simulink model "asbCubeSat.backup_210716a"  (R2020b)
settings: Solver=ode3  StartTime=0.0  StopTime=stopTime  FixedStep=CubeSatTimeStep  RelTol=1e-3  EnableMultiTasking=on
PreLoadFcn:
  | if ~builtin('license','test','Virtual_Reality_Toolbox')
  |     assignin('base','variantVisualization',0)
  | end
InitFcn:
  | if evalin('base', 'exist(''variantVisualization'',''var'')') && ...
  |         evalin('base', 'variantVisualization == 1')
  |     if ~builtin('license','checkout','Virtual_Reality_Toolbox')
  |         error(message('aeroblks_cubesat:cubesat:licenseFailAnim'));
  |     end
  | end
  | 
  | if ~evalin('base','exist(''CubeSatTimeStep'')')
  |     assignin('base','CubeSatTimeStep',1);
  | end
libraries: aerolibutil x20, aerolibconvert2 x7, simulink x3, vrlib x2, asbCubeSatEnvironmentLib x1, SignalEditorBlockLib x1, sharedutil x1, asbCubeSatActuatorsLib x1, asbCubeSatSensorsLib x1, asbCubeSatDynamicsLib x1, asbCubeSatFSWLib x1, aerolibobsolete x1
settings Model: RequirementInfo={} %GIDa_aedc6be2_fb6a_446c_8c25_10b8bc9db182  SnapshotInterval=1  EnablePacing=on  PacingRate=333  ExtModeAutoUpdateStatusClock=off  OrderedModelArguments=off  Creator=The MathWorks, Inc.  LastModifiedBy=Rodrigo.weber
settings DataIOCC: LimitDataPoints=on  SaveFormat=Array  SaveOutput=off  DSMLogging=off  SaveTime=off  ReturnWorkspaceOutputs=off
settings OptimizationCC: DefaultParameterBehavior=Inlined  OptimizeBlockIOStorage=off  BufferReuse=off  GlobalBufferReuse=off  ExpressionFolding=off  ExpressionDepthLimit=2147483647  LocalBlockOutputs=off  InitFltsAndDblsToZero=on  LifeSpan=inf  OptimizeDataStoreBuffers=off  BusAssignmentInplaceUpdate=off
settings DebuggingCC: SignalResolutionControl=TryResolveAllWithWarning  MultiTaskDSMMsg=warning  MultiTaskCondExecSysMsg=none  AssertControl=DisableAll  StateNameClashWarn=warning  PregeneratedLibrarySubsystemCodeDiagnostic=none  SFUnexpectedBacktrackingDiag=warning  SFNoUnconditionalDefaultTransitionDiag=warning  SFExecutionAtInitializationDiag=none  ArithmeticOperatorsInVariantConditions=warning
settings HardwareCC: ProdBitPerPointer=32  ProdBitPerSizeT=32  ProdBitPerPtrDiffT=32  ProdLargestAtomicFloat=None  ProdIntDivRoundTo=Undefined  ProdEndianess=Unspecified  ProdWordSize=32  ProdHWDeviceType=32-bit Generic
settings ModelReferenceCC: UpdateModelReferenceTargets=IfOutOfDate  ModelReferenceMinAlgLoopOccurrences=on  PropagateSignalLabelsOutOfModel=off
settings SFSimCC: SimUseLocalCustomCode=off
settings RTWCC: RTWUseLocalCustomCode=off
settings CodeAppCC: StateflowObjectComments=on
settings GRTTargetCC: TargetFcnLib=ansi_tfl_tmw.mat  TargetLangStandard=C89/C90 (ANSI)  CombineOutputUpdateFcns=off  GRTInterface=on
settings ConfigComp: CovMetricSettings=dw  CovSaveCumulativeToWorkspaceVar=on  CovSaveSingleToWorkspaceVar=on  CovExternalEMLEnable=off

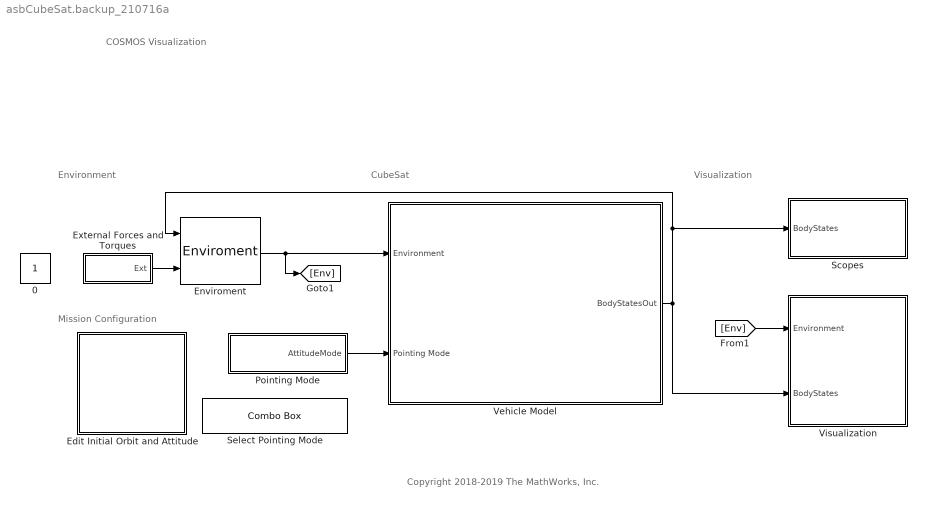
== system asbCubeSat.backup_210716a ==
  note: Visualization
  note: CubeSat
  note: Environment
  note: Copyright 2018-2019 The MathWorks, Inc.
  note: COSMOS
      | Visualization
  note: Mission Configuration
  Edit Initial Orbit and Attitude : Subsystem  mask(CubeSat Initial Conditions){sim_t0=2458488, epoch=2451545, method=Keplerian Orbital Elements, a=7086233.13, ecc=0, incl=51.7519, omega=95.2562, argp=93.4872, nu=302.9234, truelon=0, arglat=0, lonper=0, r_eci=[-649165.38524 7056435.6637 0], v_eci=[-4623.4845 -425.34309 5890.0297], r_ecef=[-7011830.8459 1024171.027 -1366.7752123], v_ecef=[-599.03035 -4093.3209 5881.6205], lla=[-0.01111806026 171.6899547 708096.1308], v_ned=[5881.6206 4136.9206 0.0068768912], euler=[0 0 0], pqr=[0 0 -0.05168], dAT=37, dUT1=-0.1193, pm=[2.141e-05 6.93e-05], dCIP=[1.014e-07 -6.81e-08], lod=0}
      mask prompts: sim_t0 "aeroblks_cubesat:cubesat:StartDate"; epoch "aeroblks_cubesat:cubesat:ECIEpoch"; method "aeroblks_cubesat:cubesat:InputMethod"; a "aeroblks_cubesat:cubesat:SemiMajorAxis"; ecc "aeroblks_cubesat:cubesat:Eccentricity"; incl "aeroblks_cubesat:cubesat:Inclination"; omega "aeroblks_cubesat:cubesat:RAAN"; argp "aeroblks_cubesat:cubesat:ArgP"; nu "aeroblks_cubesat:cubesat:TrueAnomaly"; truelon "aeroblks_cubesat:cubesat:TrueLon"; arglat "aeroblks_cubesat:cubesat:ArgLat"; lonper "aeroblks_cubesat:cubesat:LonPer"; r_eci "aeroblks_cubesat:cubesat:ECIPos"; v_eci "aeroblks_cubesat:cubesat:ECIVel"; r_ecef "aeroblks_cubesat:cubesat:ECEFPos"; v_ecef "aeroblks_cubesat:cubesat:ECEFVel"; lla "aeroblks_cubesat:cubesat:LLA"; v_ned "aeroblks_cubesat:cubesat:NEDVel"; euler "aeroblks_cubesat:cubesat:Euler"; pqr "aeroblks_cubesat:cubesat:BodyAngRates"; dAT "aeroblks_cubesat:cubesat:dTAI"; dUT1 "aeroblks_cubesat:cubesat:DUT1"; pm "aeroblks_cubesat:cubesat:DPolar"; dCIP "aeroblks_cubesat:cubesat:DCIP"; lod "aeroblks_cubesat:cubesat:DLOD"
      mask help: aeroblks_cubesat:cubesat:InitCondBlockDesc
      mask init:
      | initCond = cubeSatCallback(gcb, 'computeIC', method, sim_t0, epoch, a, ecc, incl,...
      |     omega, argp, nu, truelon, arglat, lonper, r_eci, v_eci, r_ecef, v_ecef, lla,...
      |     v_ned, euler, pqr, dAT, dUT1, pm, dCIP, lod);
      mask TypeOptions method: aeroblks_cubesat:cubesat:InputKeplerian | aeroblks_cubesat:cubesat:InputECI | aeroblks_cubesat:cubesat:InputECEF | aeroblks_cubesat:cubesat:InputLLANED
      mask Callback method: cubeSatCallback(gcb, 'handleMethod');
      mask Callback ecc: cubeSatCallback(gcb, 'handleCircularOrbit');
      mask Callback incl: cubeSatCallback(gcb, 'handleCircularOrbit');
      mask DialogControl sim_t0 Prompt: Start date [Julian date]:
      mask DialogControl sim_t0 Tooltip: aeroblks_cubesat:cubesat:StartDateTT
      mask DialogControl icTab Prompt: aeroblks_cubesat:cubesat:InitCond
      mask DialogControl epoch Prompt: Epoch of ECI frame [Julian date]:
      mask DialogControl epoch Tooltip: aeroblks_cubesat:cubesat:ECIEpochTT
      mask DialogControl Container9 Prompt: aeroblks_cubesat:cubesat:InitCondOrbit
      mask DialogControl method Prompt: Input method:
      mask DialogControl method Tooltip: aeroblks_cubesat:cubesat:InputMethodTT
      mask DialogControl a Prompt: Semi-major axis [m]:
      mask DialogControl a Tooltip: aeroblks_cubesat:cubesat:SemiMajorAxisTT
      mask DialogControl ecc Prompt: Eccentricity:
      mask DialogControl ecc Tooltip: aeroblks_cubesat:cubesat:EccentricityTT
      mask DialogControl incl Prompt: Inclination [deg]:
      mask DialogControl incl Tooltip: aeroblks_cubesat:cubesat:InclinationTT
      mask DialogControl omega Prompt: Right ascension of the ascending node [deg]:
      mask DialogControl omega Tooltip: aeroblks_cubesat:cubesat:RAANTT
      mask DialogControl argp Prompt: Argument of periapsis [deg]:
      mask DialogControl argp Tooltip: aeroblks_cubesat:cubesat:ArgPTT
      mask DialogControl nu Prompt: True anomaly [deg]:
      mask DialogControl nu Tooltip: aeroblks_cubesat:cubesat:TrueAnomalyTT
      mask DialogControl truelon Prompt: True longitude [deg] (circular equatorial):
      mask DialogControl truelon Tooltip: aeroblks_cubesat:cubesat:TrueLonTT
      mask DialogControl arglat Prompt: Argument of latitude [deg] (circular inclined):
      mask DialogControl arglat Tooltip: aeroblks_cubesat:cubesat:ArgLatTT
      mask DialogControl lonper Prompt: Longitude of periapsis [deg] (elliptical equatorial):
      mask DialogControl lonper Tooltip: aeroblks_cubesat:cubesat:LonPerTT
      mask DialogControl r_eci Prompt: ECI position vector [m]:
      mask DialogControl r_eci Tooltip: aeroblks_cubesat:cubesat:ECIPosTT
      mask DialogControl v_eci Prompt: ECI velocity vector [m/s]:
      mask DialogControl v_eci Tooltip: aeroblks_cubesat:cubesat:ECIVelTT
      mask DialogControl r_ecef Prompt: ECEF position vector [m]:
      mask DialogControl r_ecef Tooltip: aeroblks_cubesat:cubesat:ECEFPosTT
      mask DialogControl v_ecef Prompt: ECEF velocity vector [m/s]:
      mask DialogControl v_ecef Tooltip: aeroblks_cubesat:cubesat:ECEFVelTT
      mask DialogControl lla Prompt: Geodetic latitude, longitude, altitude [deg, deg, m]:
      mask DialogControl lla Tooltip: aeroblks_cubesat:cubesat:LLATT
      mask DialogControl v_ned Prompt: NED velocity vector [m/s]:
      mask DialogControl v_ned Tooltip: aeroblks_cubesat:cubesat:NEDVelTT
      mask DialogControl Container11 Prompt: aeroblks_cubesat:cubesat:InitCondAttitude
      mask DialogControl euler Prompt: <html>Initial Euler angles (roll, pitch, yaw) [deg]:</html>
      mask DialogControl euler Tooltip: aeroblks_cubesat:cubesat:EulerTT
      mask DialogControl pqr Prompt: Initial body angular rates [deg/s]:
      mask DialogControl pqr Tooltip: aeroblks_cubesat:cubesat:BodyAngRatesTT
      mask DialogControl epTab Prompt: aeroblks_cubesat:cubesat:EOPTab
      mask DialogControl dAT Prompt: Difference between TAI and UTC [sec]:
      mask DialogControl dAT Tooltip: aeroblks_cubesat:cubesat:dTAITT
      mask DialogControl dUT1 Prompt: Difference between UTC and UT1 [sec]:
      mask DialogControl dUT1 Tooltip: aeroblks_cubesat:cubesat:DUT1TT
      mask DialogControl pm Prompt: Polar displacement [deg deg]:
      mask DialogControl pm Tooltip: aeroblks_cubesat:cubesat:DPolarTT
      mask DialogControl dCIP Prompt: CIP adjustment [deg deg]:
      mask DialogControl dCIP Tooltip: aeroblks_cubesat:cubesat:DCIPTT
      mask DialogControl lod Prompt: Excess length of day [sec]:
      mask DialogControl lod Tooltip: aeroblks_cubesat:cubesat:DLODTT
      mask Display:
      | text(.1, .9, [' a = ' sprintf('%.1f', str2double(get_param(gcb, 'a'))) ' m'],'horizontalAlignment','left','texmode','on');
      | text(.1, .75, [' e = ' get_param(gcb, 'ecc')],'horizontalAlignment','left','texmode', 'on')
      | text(.1, .6, ['  i = ' get_param(gcb, 'incl') '\circ'],'horizontalAlignment','left','texmode', 'on')
      | text(.1, .45, ['\Omega = ' get_param(gcb, 'omega') '\circ'],'horizontalAlignment','left','texmode', 'on')
      | text(.1, .3, ['\omega = ' get_param(gcb, 'argp') '\circ'],'horizontalAlignment','left','texmode', 'on')
      | text(.1, .15, [' \nu = ' get_param(gcb, 'nu') '\circ'],'horizontalAlignment','left','texmode', 'on')
  Enviroment : asbCubeSatEnvironmentLib/Enviroment  SystemSampleTime=-1  VariantActivationTime=update diagram  Latency=0  AutoFrameSizeCalculation=off
  "External Forces and Torques " : Subsystem
  Pointing Mode : Subsystem
  Scopes : Subsystem  VariantControl=visOff
  Select Pointing Mode : ComboBox  LabelPosition=Hide  SelectedLabel=Nadir Pointing (Earth)
      settings: Values={{'Standby', 'Nadir Pointing (Earth)', 'Sun Tracking', 'Custom Schedule'}, [0 1 2 3]}
  Vehicle Model : Subsystem
      mask Display: image('CubeSatVehicle.PNG');
  Visualization : Subsystem  Variant=on  mask(Set Animation Properties){visSampleTime=5, cubesatSize=2e5, showAntenna=on, antennaHeight=1e6, antennaHalfAngle=25}
      mask prompts: visSampleTime "aeroblks_cubesat:cubesat:AnimSampleTime"; cubesatSize "aeroblks_cubesat:cubesat:MdlSize"; showAntenna "aeroblks_cubesat:cubesat:ShowCone"; antennaHeight "aeroblks_cubesat:cubesat:ConeHeight"; antennaHalfAngle "aeroblks_cubesat:cubesat:ConeAngle"
      mask help: aeroblks_cubesat:cubesat:VisBlockDesc
      mask Callback showAntenna:
      | if evalin('base', 'exist(''variantVisualization'',''var'')') ...
      |     && evalin('base', 'variantVisualization == 1') ...
      |     && builtin('license','test','Virtual_Reality_Toolbox')
      | 
      |     enable = get_param(gcb,'MaskEnables');
      |     if strcmp(get_param(gcb, 'showAntenna'), 'off')
      |         enable(4:5) = {'off'};
      |     else
      |         enable(4:5) = {'on'};
      |     end
      |     set_param(gcb,'MaskEnables', enable);
      |     clear enable
      | end
      mask DialogControl vrOpenBtn Prompt: aeroblks_cubesat:cubesat:AnimOpenBtn
      mask DialogControl vrOpenBtn Callback:
      | if builtin('license','checkout','Virtual_Reality_Toolbox')
      |     vrmfunc('FnOpen',getSimulinkBlockHandle([gcb '/Virtual Reality World/VR Sink']));
      | end
      mask DialogControl visSampleTime Prompt: Animation refresh rate:
      mask DialogControl visSampleTime Tooltip: aeroblks_cubesat:cubesat:AnimSampleTimeTT
      mask DialogControl cubesatSize Prompt: CubeSat display size [m]:
      mask DialogControl cubesatSize Tooltip: aeroblks_cubesat:cubesat:MdlSizeTT
      mask DialogControl Container3 Prompt: aeroblks_cubesat:cubesat:AntennaPropArea
      mask DialogControl showAntenna Prompt: Show antenna cone in animation
      mask DialogControl showAntenna Tooltip: aeroblks_cubesat:cubesat:ShowConeTT
      mask DialogControl antennaHeight Prompt: Antenna cone height [m]:
      mask DialogControl antennaHeight Tooltip: aeroblks_cubesat:cubesat:ConeHeightTT
      mask DialogControl antennaHalfAngle Prompt: Antenna cone half angle [deg]:
      mask DialogControl antennaHalfAngle Tooltip: aeroblks_cubesat:cubesat:ConeAngleTT
  0 : Constant  IOType=siggen
  wires:
  Enviroment/1 -> [Env], Vehicle Model/1(Environment)
  "External Forces and Torques "/1(Ext) -> Enviroment/2
  Vehicle Model/1(BodyStatesOut) -> Visualization/2(BodyStates), Scopes/1(BodyStates), Enviroment/1
  Pointing Mode/1(AttitudeMode) -> Vehicle Model/2(Pointing Mode)
  [Env] -> Visualization/1(Environment)

== system asbCubeSat.backup_210716a/Edit Initial Orbit and Attitude ==

== system asbCubeSat.backup_210716a/External Forces and Torques  ==
  Forces_Body : Constant  Value=[0 0 0]
  Mux : Mux  RequirementInfo={} %GIDa_ef4ca723_4eef_40f8_bb1e_99de60d2b248  Inputs=2
  Torques_Body : Constant  Value=[0 0 0]
  Ext : Outport  RequirementInfo={} %GIDa_0f078eca_6127_499d_b81c_658503a40261  VectorParamsAs1DForOutWhenUnconnected=off
  wires:
  Forces_Body/1 -> Mux/1
  Torques_Body/1 -> Mux/2
  Mux/1 -> Ext/1

== system asbCubeSat.backup_210716a/Pointing Mode ==
  note: Modes:
      | 0 = Off
      | 1 = Earth (Nadir)
      | 2 = Sun
  Mode : Constant  SampleTime=-1
  Multiport Switch : MultiPortSwitch  DataPortOrder=Specify indices  DataPortIndices={3, [0,1,2]}  DiagnosticForDefault=None
  Signal Editor : SignalEditorBlockLib/Signal Editor  FileName=SignalEditorPointing.mat  ActiveScenario=PointingScenario  ActiveSignal=PointingMode  IsBus=off  OutputBusObjectStr=Bus: BusObject  SampleTime=0  Interpolate=off  ZeroCross=off  OutputAfterFinalValue=Setting to zero  Unit=inherit  PreserveSignalName=on
  AttitudeMode : Outport  VectorParamsAs1DForOutWhenUnconnected=off
  wires:
  Signal Editor/1 -> Multiport Switch/2
  Mode/1 -> Multiport Switch/1, Multiport Switch/3
  Multiport Switch/1 -> AttitudeMode/1

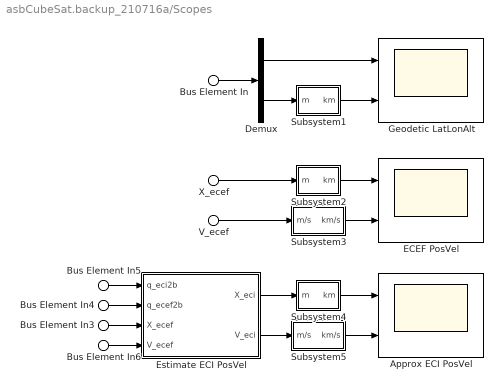
== system asbCubeSat.backup_210716a/Scopes ==
  Bus Element In : Inport  PortName=BodyStates  Element=LatLonAlt
  X_ecef : Inport  PortName=BodyStates  Element=X_ecef
  Bus Element In3 : Inport  PortName=BodyStates  Element=X_ecef
  V_ecef : Inport  PortName=BodyStates  Element=V_ecef
  Bus Element In6 : Inport  PortName=BodyStates  Element=V_ecef
  Bus Element In4 : Inport  PortName=BodyStates  Element=q_ecef2b
  Bus Element In5 : Inport  PortName=BodyStates  Element=q_eci2b
  Approx ECI PosVel : Scope  NumInputPorts=2
  Demux : Demux  Outputs=[2 1]
  ECEF PosVel : Scope  NumInputPorts=2
  Estimate ECI PosVel : Subsystem
  Geodetic LatLonAlt : Scope  NumInputPorts=2
  Subsystem1 : Subsystem
  Subsystem2 : Subsystem
  Subsystem3 : Subsystem
  Subsystem4 : Subsystem
  Subsystem5 : Subsystem
  wires:
  Bus Element In/1 -> Demux/1
  Demux/1 -> Geodetic LatLonAlt/1
  Demux/2 -> Subsystem1/1(m)
  X_ecef/1 -> Subsystem2/1(m)
  V_ecef/1 -> Subsystem3/1(m/s)
  Estimate ECI PosVel/1(X_eci) -> Subsystem4/1(m)
  Estimate ECI PosVel/2(V_eci) -> Subsystem5/1(m/s)
  Bus Element In5/1 -> Estimate ECI PosVel/1(q_eci2b)
  Bus Element In4/1 -> Estimate ECI PosVel/2(q_ecef2b)
  Bus Element In3/1 -> Estimate ECI PosVel/3(X_ecef)
  Bus Element In6/1 -> Estimate ECI PosVel/4(V_ecef)
  Subsystem1/1(km) -> Geodetic LatLonAlt/2
  Subsystem2/1(km) -> ECEF PosVel/1
  Subsystem3/1(km/s) -> ECEF PosVel/2
  Subsystem4/1(km) -> Approx ECI PosVel/1
  Subsystem5/1(km/s) -> Approx ECI PosVel/2

== system asbCubeSat.backup_210716a/Vehicle Model ==
  note: Flight Software
  note: Plant Model
  Environment : Inport
  Pointing Mode : Inport  Port=2
  Vehicle Control Actuators : asbCubeSatActuatorsLib/Vehicle Control Actuators  SystemSampleTime=-1  VariantActivationTime=update diagram  Latency=0  AutoFrameSizeCalculation=off
  Vehicle Control Sensors : asbCubeSatSensorsLib/Vehicle Control Sensors  SystemSampleTime=-1  VariantActivationTime=update diagram  Latency=0  AutoFrameSizeCalculation=off
  Vehicle Dynamics : asbCubeSatDynamicsLib/Vehicle Dynamics  SystemSampleTime=-1  VariantActivationTime=update diagram  Latency=0  AutoFrameSizeCalculation=off
  Vehicle Flight Software : asbCubeSatFSWLib/Vehicle Flight Software  SystemSampleTime=-1  VariantActivationTime=update diagram  Latency=0  AutoFrameSizeCalculation=off
  BodyStatesOut : Outport  OutDataTypeStr=Bus: StatesOutBus  VectorParamsAs1DForOutWhenUnconnected=off
  wires:
  Vehicle Dynamics/1 -> Vehicle Control Sensors/1, BodyStatesOut/1
  Pointing Mode/1 -> Vehicle Flight Software/1
  Vehicle Control Sensors/1 -> Vehicle Flight Software/3
  Vehicle Control Actuators/1 -> Vehicle Dynamics/1
  Vehicle Control Actuators/2 -> Vehicle Dynamics/2
  Vehicle Flight Software/1 -> Vehicle Control Actuators/1
  Environment/1 -> Vehicle Dynamics/3, Vehicle Flight Software/2

== system asbCubeSat.backup_210716a/Visualization ==
  Environment : Inport
  BodyStates : Inport  RequirementInfo={} %GIDa_d1e0371a_f352_4707_a071_6ff04189e700  Port=2
  No Visualization : Subsystem  VariantControl=visOff
  Virtual Reality World : Subsystem  VariantControl=visSL3D

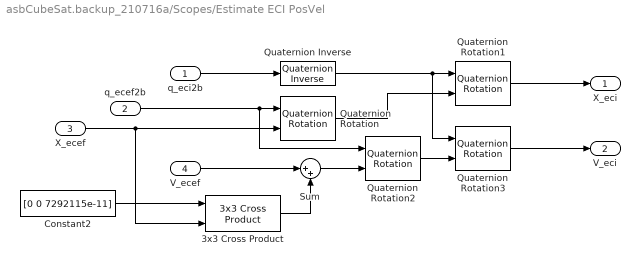
== system asbCubeSat.backup_210716a/Scopes/Estimate ECI PosVel ==
  q_eci2b : Inport
  q_ecef2b : Inport  Port=2
  X_ecef : Inport  Port=3
  V_ecef : Inport  Port=4
  3x3 Cross Product : sharedutil/3x3 Cross Product  aMode=aMode
      settings: SourceProductBaseCode=AE,PW,MT,UV,VE,VP
  Constant2 : Constant  RequirementInfo={} %GIDa_2ba99f61_3734_437b_bb66_1284a91b5056  Value=[0 0 7292115e-11]
  Quaternion Inverse : aerolibutil/Quaternion Inverse
  Quaternion Rotation{,1..3} (4 alike) : aerolibutil/Quaternion Rotation
  Sum : Sum  Inputs=|++
  X_eci : Outport  VectorParamsAs1DForOutWhenUnconnected=off
  V_eci : Outport  Port=2  VectorParamsAs1DForOutWhenUnconnected=off
  wires:
  Sum/1 -> Quaternion Rotation2/2
  3x3 Cross Product/1 -> Sum/2
  V_ecef/1 -> Sum/1
  Quaternion Rotation/1 -> Quaternion Rotation1/2
  q_ecef2b/1 -> Quaternion Rotation/1, Quaternion Rotation2/1
  Quaternion Inverse/1 -> Quaternion Rotation3/1, Quaternion Rotation1/1
  Constant2/1 -> 3x3 Cross Product/1
  Quaternion Rotation2/1 -> Quaternion Rotation3/2
  q_eci2b/1 -> Quaternion Inverse/1
  Quaternion Rotation1/1 -> X_eci/1
  X_ecef/1 -> 3x3 Cross Product/2, Quaternion Rotation/2
  Quaternion Rotation3/1 -> V_eci/1

== system asbCubeSat.backup_210716a/Scopes/Subsystem1 ==
  m : Inport  Unit=m
  Unit Conversion : UnitConversion
  km : Outport  Unit=km  VectorParamsAs1DForOutWhenUnconnected=off
  wires:
  m/1 -> Unit Conversion/1
  Unit Conversion/1 -> km/1

== system asbCubeSat.backup_210716a/Scopes/Subsystem2 ==
  m : Inport  Unit=m
  Unit Conversion : UnitConversion
  km : Outport  Unit=km  VectorParamsAs1DForOutWhenUnconnected=off
  wires:
  Unit Conversion/1 -> km/1
  m/1 -> Unit Conversion/1

== system asbCubeSat.backup_210716a/Scopes/Subsystem3 ==
  m/s : Inport  Unit=m/s
  Unit Conversion : UnitConversion
  km/s : Outport  Unit=km/s  VectorParamsAs1DForOutWhenUnconnected=off
  wires:
  m/s/1 -> Unit Conversion/1
  Unit Conversion/1 -> km/s/1

== system asbCubeSat.backup_210716a/Scopes/Subsystem4 ==
  m : Inport  Unit=m
  Unit Conversion : UnitConversion
  km : Outport  Unit=km  VectorParamsAs1DForOutWhenUnconnected=off
  wires:
  Unit Conversion/1 -> km/1
  m/1 -> Unit Conversion/1

== system asbCubeSat.backup_210716a/Scopes/Subsystem5 ==
  m/s : Inport  Unit=m/s
  Unit Conversion : UnitConversion
  km/s : Outport  Unit=km/s  VectorParamsAs1DForOutWhenUnconnected=off
  wires:
  m/s/1 -> Unit Conversion/1
  Unit Conversion/1 -> km/s/1

== system asbCubeSat.backup_210716a/Visualization/No Visualization ==
  BodyStates : Inport
  Environment : Inport  Port=2
  Terminator2 : Terminator
      settings: RequirementInfo={} %GIDa_803f6fff_5423_4e6f_a9df_7d3b0fb0a1d4
  Terminator3 : Terminator
      settings: RequirementInfo={} %GIDa_5d360e88_5b3d_45e7_ae99_5d46a57676c9
  wires:
  Environment/1 -> Terminator2/1
  BodyStates/1 -> Terminator3/1

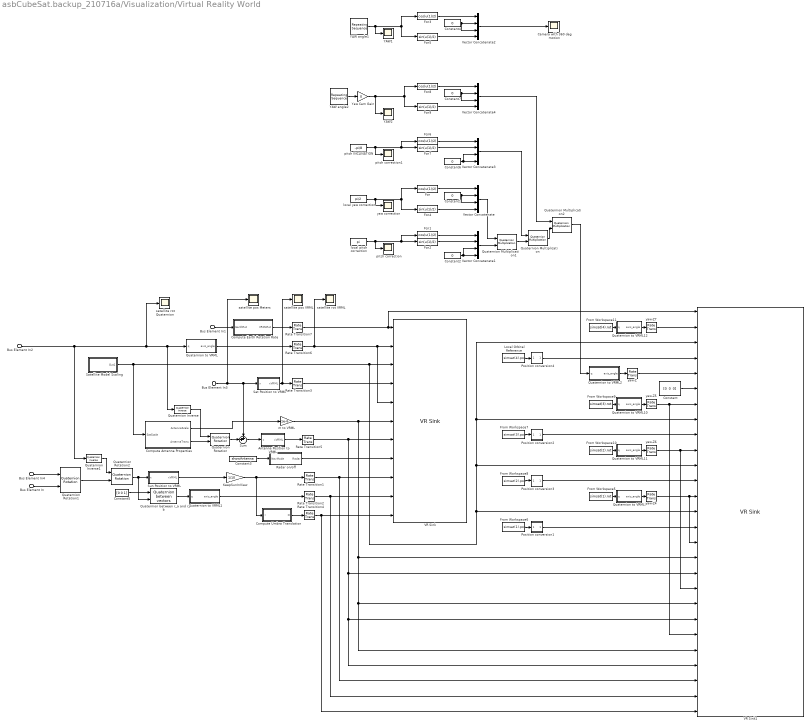
== system asbCubeSat.backup_210716a/Visualization/Virtual Reality World ==
  Bus Element In3 : Inport  PortName=BodyStates  Element=X_ecef
  Bus Element In2 : Inport  PortName=BodyStates  Element=q_ecef2b
  Bus Element In4 : Inport  PortName=BodyStates  Element=q_eci2b
  Bus Element In : Inport  Port=2  PortName=Environment  Element=x_sun_eci
  Bus Element In1 : Inport  Port=2  PortName=Environment  Element=earthAngRate
  Antenna Position to VRML : Subsystem
  Camera with 360 deg motion : Scope
  Compute Antenna Properties : Subsystem
  Compute Earth Rotation Rate : Subsystem
  Compute Umbra Translation : Subsystem
  Constant : Constant  Value="[0  0  0]"
  Constant{1..2,4,6..7} (5 alike) : Constant  Value=0
  Constant3 : Constant  Value=showAntenna
  Constant5 : Constant  Value=[0 0 1]
  Fcn{,1,3,6,8} (5 alike) : Fcn  Expr=cos(u(1)/2)
  Fcn{2,4..5,7,9} (5 alike) : Fcn  Expr=sin(u(1)/2)
  From Workspace10 : FromWorkspace  VariableName=simsat(2).rot
  From Workspace11 : FromWorkspace  VariableName=simsat(4).rot
  From Workspace5 : FromWorkspace  VariableName=simsat(1).rot
  From Workspace6 : FromWorkspace  VariableName=simsat(1).pos
  From Workspace7 : FromWorkspace  VariableName=simsat(3).pos
  From Workspace8 : FromWorkspace  VariableName=simsat(2).pos
  From Workspace9 : FromWorkspace  VariableName=simsat(3).rot
  KeepSunInView : Gain  Gain=1/10
  "Local Orbital Reference " : FromWorkspace  VariableName=simsat(4).pos
  Position conversion4 : Subsystem
  Position conversion1 : Subsystem
  Position conversion2 : Subsystem
  Position conversion3 : Subsystem
  Quaternion Inverse : aerolibutil/Quaternion Inverse
  Quaternion Inverse1 : aerolibutil/Quaternion Inverse
  Quaternion Multiplication : aerolibutil/Quaternion Multiplication
  Quaternion Multiplication1 : aerolibutil/Quaternion Multiplication
  Quaternion Multiplication2 : aerolibutil/Quaternion Multiplication
  Quaternion Rotation : aerolibutil/Quaternion Rotation
  Quaternion Rotation1 : aerolibutil/Quaternion Rotation
  Quaternion Rotation2 : aerolibutil/Quaternion Rotation
  Quaternion between r_a and r_b : aerolibattitudesys/Quaternion between vectors
      settings: SourceProductBaseCode=AERO_CUBESAT
  Quaternion to VRML : Subsystem
  Quaternion to VRML1 : Subsystem
  Quaternion to VRML10 : Subsystem
  Quaternion to VRML11 : Subsystem
  Quaternion to VRML12 : Subsystem
  Quaternion to VRML2 : Subsystem
  Quaternion to VRML9 : Subsystem
  Radar on/off : Subsystem
  Rate Transition{1..7} (7 alike) : RateTransition
  Sat Position to VRML : Subsystem
  Satellite Model Scaling : Subsystem
  Sum : Sum  Inputs=++|
  Sun Position to VRML : Subsystem
  VR Sink : vrlib/VR Sink  InstantiateOnLoad=on  SampleTime=visSampleTime  ViewEnable=on  RemoteChange=off  RemoteView=off  FieldsWritten=Earth.rotation.4.1.1.double#Satellite.rotation.4.1.1.double#Satellite.scale.3.1.1.double#Satellite.translation.3.1.1.double#AntennaCone.rotation.4.1.1.double#AntennaCone.scale.3.1.1.double#AntennaCone.translation.3.1.1.double#AntennaMaterial.transparency.1.1.1.double#Sun.translation.3.1.1.double#Umbra.rotation.4.1.1.double#Umbra.translation.3.1.1.double  WorldFileName=cubesatAnim.wrl  WorldDescription=CubeSat Orbit Animation  AutoView=off  VideoDimensions=[]  AllowVariableSize=off
  VR Sink1 : vrlib/VR Sink  InstantiateOnLoad=on  SampleTime=visSampleTime  ViewEnable=on  RemoteChange=off  RemoteView=off  FieldsWritten=Earth.rotation.4.1.1.double#SatelliteReference.rotation.4.1.1.double#SatelliteReference.scale.3.1.1.double#SatelliteReference.translation.3.1.1.double#FollowReference.rotation.4.1.1.double#FollowReference.translation.3.1.1.double#Satellite3.rotation.4.1.1.double#Satellite3.scale.3.1.1.double#Satellite3.translation.3.1.1.double#Satellite2.rotation.4.1.1.double#Satellite2.scale.3.1.1.double#Satellite2.translation.3.1.1.double#Satellite1.rotation.4.1.1.double#Satellite1.scale.3.1.1.double#Satellite1.translation.3.1.1.double#AntennaCone1.rotation.4.1.1.double#AntennaCone1.scale.3.1.1.double#AntennaCone1.translation.3.1.1.double#AntennaCone2.rotation.4.1.1.double#AntennaCone2.scale.3.1.1.double#AntennaCone2.translation.3.1.1.double#AntennaCone3.rotation.4.1.1.double#AntennaCone3.scale.3.1.1.double#AntennaCone3.translation.3.1.1.double#Sun.translation.3.1.1.double#Umbra.rotation.4.1.1.double#Umbra.translation.3.1.1.double  WorldFileName=cosmosSimulation.x3d  WorldDescription=COSMOS Visualization  AutoView=on  VideoDimensions=[]  AllowVariableSize=off  FigureProperties="{'Position', 'Name', 'Viewpoint', 'CameraBound', 'CameraDirection', 'CameraPosition', 'CameraUpVector', 'ZoomFactor', 'Antialiasing', 'Headlight', 'Lighting', 'NavPanel', 'Sound', 'StatusBar', 'Stereo3D', 'Stereo3DCameraOffset', 'Stereo3DHIT', 'ToolBar', 'Textures', 'Transparency', 'Triad', 'Wireframe', 'NavZones', 'NavMode', 'NavSpeed', 'CaptureFileFormat', 'CaptureFileName', 'Record2DCompressMethod', 'Record2DCompressQuality', 'Record2D', 'Record2DFileName', 'Record2DFPS'; [2.0000000000000000e+00   8.4000000000000000e+01   9.5800000000000000e+02   8.6300000000000000e+02], 'COSMOS Visualization', 'Follow Local-Ref', 'on', [0.0000000000000000e+00   0.0000000000000000e+00  -1.0000000000000000e+00], [0.0000000000000000e+00   0.0000000000000000e+00   1.0000000000000000e+01], [0.0000000000000000e+00   1.0000000000000000e+00   0.0000000000000000e+00], [1.0000000000000000e+00], 'on', 'on', 'on', 'halfbar', 'on', 'on', 'off', [1.0000000149011612e-01], [0.0000000000000000e+00], 'on', 'on', 'on', 'none', 'off', 'off', 'examine', 'normal', 'tif', '%f_anim_%n.tif', 'auto', [7.5000000000000000e+01], 'on', '..\\recordings\\cosmos-animation-%n.avi', [3.0000000000000000e+01]}"
  Vector Concatenate{,1..4} (5 alike) : Concatenate  NumInputs=4
  YAW angle1 : simulink/Sources/Repeating Sequence  rep_seq_t=[0 0.5e4]  rep_seq_y=[0 2*pi]
  YAW angle2 : simulink/Sources/Repeating Sequence  rep_seq_t="[0 0.5e4 1e4 1.5e4 2e4 2.5e4 3e4  3.5e4  4e4]"  rep_seq_y="[0 pi/2   pi/2  0       0     -pi/2 -pi/2  0     0]"
  YAW1 : Scope
  YAW2 : Scope
  Yaw Cam Gain : Gain  Gain=0
  local pitch correction : Constant  Value=pi
  local yaw correction : Constant  Value=pi/2
  m to VRML : Gain  Gain=1e-6
  pitch INCLINATION : Constant  Value=-pi/8
  pitch correction : Scope
  pitch correction1 : Scope
  satellite pos Meters : Scope
  satellite pos VRML : Scope
  satellite rot Quaternion : Scope
  satellite rot VRML : Scope
  yaw correction : Scope
  yaw-Z{,4..7} (5 alike) : RateTransition
  wires:
  Bus Element In2/1 -> satellite rot Quaternion/1, Quaternion to VRML/1(q), Quaternion Inverse/1, Quaternion Inverse1/1
  Constant3/1 -> Radar on/off/1(NavMode)
  Bus Element In3/1 -> satellite pos Meters/1, Sat Position to VRML/1(x), Sum/1
  Quaternion Inverse/1 -> Quaternion Rotation/1
  Sum/1 -> Antenna Position to VRML/1(x)
  Quaternion Rotation/1 -> Sum/2
  Quaternion Rotation2/1 -> Sun Position to VRML/1(x), Quaternion between r_a and r_b/2
  Quaternion Rotation1/1 -> Quaternion Rotation2/2
  Quaternion Inverse1/1 -> Quaternion Rotation2/1
  Sun Position to VRML/1(xVRML) -> KeepSunInView/1
  Quaternion between r_a and r_b/1 -> Quaternion to VRML1/1(q)
  Constant5/1 -> Quaternion between r_a and r_b/1
  Antenna Position to VRML/1(xVRML) -> Rate Transition5/1
  Compute Earth Rotation Rate/1(VRMLRot) -> Rate Transition7/1
  Sat Position to VRML/1(xVRML) -> satellite pos VRML/1, Rate Transition3/1
  Radar on/off/1(Radar) -> VR Sink/8
  Quaternion to VRML1/1(axis_angle) -> Rate Transition2/1
  KeepSunInView/1 -> Compute Umbra Translation/1(I), Rate Transition1/1
  Compute Umbra Translation/1(O) -> Rate Transition4/1
  Compute Antenna Properties/1(AntennaScale) -> m to VRML/1
  Compute Antenna Properties/2(AntennaTrans) -> Quaternion Rotation/2
  Bus Element In4/1 -> Quaternion Rotation1/1
  Bus Element In/1 -> Quaternion Rotation1/2
  Rate Transition2/1 -> VR Sink/10, VR Sink1/26
  Bus Element In1/1 -> Compute Earth Rotation Rate/1(EarthRot)
  Quaternion to VRML/1(axis_angle) -> Rate Transition6/1
  Rate Transition7/1 -> VR Sink/1, VR Sink1/1
  Rate Transition6/1 -> VR Sink/2, VR Sink/5, satellite rot VRML/1
  Rate Transition5/1 -> VR Sink1/24, VR Sink1/21, VR Sink1/18, VR Sink/7
  m to VRML/1 -> VR Sink1/20, VR Sink1/23, VR Sink1/17, VR Sink/6
  Rate Transition3/1 -> VR Sink/4
  Rate Transition1/1 -> VR Sink/9, VR Sink1/25
  Rate Transition4/1 -> VR Sink/11, VR Sink1/27
  Quaternion to VRML9/1(axis_angle) -> yaw-Z4/1
  From Workspace5/1 -> Quaternion to VRML9/1(q)
  From Workspace6/1 -> Position conversion1/1(In1)
  From Workspace7/1 -> Position conversion2/1(In1)
  From Workspace8/1 -> Position conversion3/1(In1)
  From Workspace9/1 -> Quaternion to VRML10/1(q)
  Quaternion to VRML10/1(axis_angle) -> yaw-Z5/1
  From Workspace10/1 -> Quaternion to VRML11/1(q)
  Quaternion to VRML11/1(axis_angle) -> yaw-Z6/1
  "Local Orbital Reference "/1 -> Position conversion4/1(In1)
  From Workspace11/1 -> Quaternion to VRML12/1(q)
  Quaternion to VRML12/1(axis_angle) -> yaw-Z7/1
  Fcn4/1 -> Vector Concatenate/4
  local yaw correction/1 -> yaw correction/1, Fcn4/1, Fcn/1
  Fcn/1 -> Vector Concatenate/1
  Constant1/1 -> Vector Concatenate/2, Vector Concatenate/3
  Quaternion to VRML2/1(axis_angle) -> yaw-Z/1
  Fcn2/1 -> Vector Concatenate1/2
  Constant2/1 -> Vector Concatenate1/3, Vector Concatenate1/4
  local pitch correction/1 -> pitch correction/1, Fcn2/1, Fcn1/1
  Fcn1/1 -> Vector Concatenate1/1
  Fcn3/1 -> Vector Concatenate2/1
  Constant4/1 -> Vector Concatenate2/2, Vector Concatenate2/3
  Fcn5/1 -> Vector Concatenate2/4
  YAW angle1/1 -> YAW1/1, Fcn5/1, Fcn3/1
  Vector Concatenate1/1 -> Quaternion Multiplication1/2
  Vector Concatenate/1 -> Quaternion Multiplication1/1
  Quaternion Multiplication2/1 -> Quaternion to VRML2/1(q)
  Fcn7/1 -> Vector Concatenate3/2
  Constant6/1 -> Vector Concatenate3/3, Vector Concatenate3/4
  Fcn6/1 -> Vector Concatenate3/1
  pitch INCLINATION/1 -> pitch correction1/1, Fcn7/1, Fcn6/1
  Quaternion Multiplication1/1 -> Quaternion Multiplication/2
  Vector Concatenate3/1 -> Quaternion Multiplication/1
  Constant7/1 -> Vector Concatenate4/2, Vector Concatenate4/3
  Fcn9/1 -> Vector Concatenate4/4
  YAW angle2/1 -> Yaw Cam Gain/1
  Fcn8/1 -> Vector Concatenate4/1
  Quaternion Multiplication/1 -> Quaternion Multiplication2/2
  Vector Concatenate4/1 -> Quaternion Multiplication2/1
  yaw-Z7/1 -> VR Sink1/2
  Satellite Model Scaling/1(Out1) -> VR Sink/3, VR Sink1/14, VR Sink1/3, VR Sink1/8, VR Sink1/11, Compute Antenna Properties/1(SatScale)
  Position conversion4/1(Out1) -> VR Sink1/4
  yaw-Z/1 -> VR Sink1/5
  Constant/1 -> VR Sink1/6
  yaw-Z5/1 -> VR Sink1/7, VR Sink1/22
  Position conversion2/1(Out1) -> VR Sink1/9
  yaw-Z6/1 -> VR Sink1/10, VR Sink1/19
  Position conversion3/1(Out1) -> VR Sink1/12
  yaw-Z4/1 -> VR Sink1/13, VR Sink1/16
  Position conversion1/1(Out1) -> VR Sink1/15
  Vector Concatenate2/1 -> Camera with 360 deg motion/1
  Yaw Cam Gain/1 -> Fcn9/1, Fcn8/1, YAW2/1

== system asbCubeSat.backup_210716a/Visualization/Virtual Reality World/Antenna Position to VRML ==
  x : Inport
  ECEF to VRML : Subsystem
  Length Conversion : aerolibconvert2/Length Conversion  IU=m  OU=km
  km to VRML units : Gain  Gain=1/1000
  xVRML : Outport  VectorParamsAs1DForOutWhenUnconnected=off
  wires:
  Length Conversion/1 -> km to VRML units/1
  km to VRML units/1 -> ECEF to VRML/1(M)
  x/1 -> Length Conversion/1
  ECEF to VRML/1(VR) -> xVRML/1

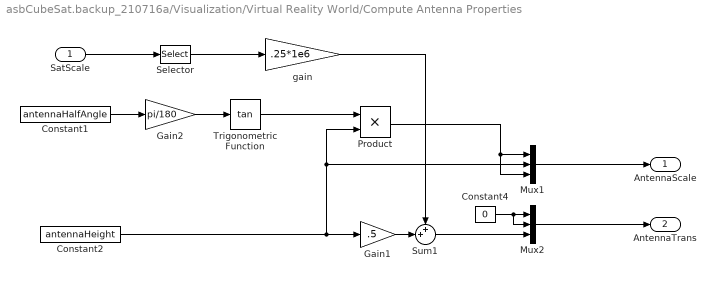
== system asbCubeSat.backup_210716a/Visualization/Virtual Reality World/Compute Antenna Properties ==
  SatScale : Inport
  Constant1 : Constant  Value=antennaHalfAngle
  Constant2 : Constant  Value=antennaHeight
  Constant4 : Constant  Value=0
  Gain1 : Gain  Gain=.5
  Gain2 : Gain  Gain=pi/180
  Mux1 : Mux  Inputs=3
  Mux2 : Mux  Inputs=3
  Product : Product
  Selector : Selector  InputPortWidth=3  IndexOptions=Index vector (dialog)  Indices=1  OutputSizes=1
  Sum1 : Sum  Inputs=++|
  Trigonometric Function : Trigonometry  Operator=tan
  gain : Gain  Gain=.25*1e6
  AntennaScale : Outport  VectorParamsAs1DForOutWhenUnconnected=off
  AntennaTrans : Outport  Port=2  VectorParamsAs1DForOutWhenUnconnected=off
  wires:
  Gain2/1 -> Trigonometric Function/1
  Constant4/1 -> Mux2/1, Mux2/2
  Sum1/1 -> Mux2/3
  Constant2/1 -> Gain1/1, Mux1/2, Product/2
  gain/1 -> Sum1/1
  Constant1/1 -> Gain2/1
  Product/1 -> Mux1/3, Mux1/1
  Gain1/1 -> Sum1/2
  Trigonometric Function/1 -> Product/1
  Mux2/1 -> AntennaTrans/1
  Mux1/1 -> AntennaScale/1
  SatScale/1 -> Selector/1
  Selector/1 -> gain/1

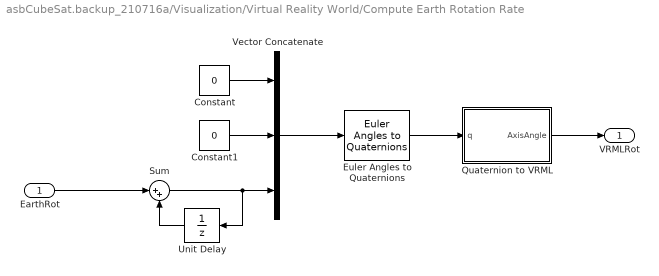
== system asbCubeSat.backup_210716a/Visualization/Virtual Reality World/Compute Earth Rotation Rate ==
  EarthRot : Inport
  Constant : Constant  Value=0
  Constant1 : Constant  Value=0
  Euler Angles to Quaternions : aerolibobsolete/Euler Angles to Quaternions
      settings: SourceProductBaseCode=AE
  Quaternion to VRML : Subsystem
  Sum : Sum  Inputs=|++
  Unit Delay : UnitDelay  SampleTime=-1  HasFrameUpgradeWarning=on
  Vector Concatenate : Concatenate  NumInputs=3
  VRMLRot : Outport  VectorParamsAs1DForOutWhenUnconnected=off
  wires:
  EarthRot/1 -> Sum/1
  Unit Delay/1 -> Sum/2
  Sum/1 -> Vector Concatenate/3, Unit Delay/1
  Constant/1 -> Vector Concatenate/1
  Constant1/1 -> Vector Concatenate/2
  Vector Concatenate/1 -> Euler Angles to Quaternions/1
  Euler Angles to Quaternions/1 -> Quaternion to VRML/1(q)
  Quaternion to VRML/1(AxisAngle) -> VRMLRot/1

== system asbCubeSat.backup_210716a/Visualization/Virtual Reality World/Compute Umbra Translation ==
  I : Inport
  Add : Sum
  ConeHalfLength : Gain  Gain=692
  InvertSunPosECEF : Gain  Gain=-1
  unitVec : Subsystem
  O : Outport  VectorParamsAs1DForOutWhenUnconnected=off
  wires:
  ConeHalfLength/1 -> Add/2
  I/1 -> InvertSunPosECEF/1
  Add/1 -> O/1
  InvertSunPosECEF/1 -> unitVec/1(I), Add/1
  unitVec/1(O) -> ConeHalfLength/1

== system asbCubeSat.backup_210716a/Visualization/Virtual Reality World/Position conversion4 ==
  In1 : Inport
  Rate Transition11 : RateTransition
  Sat Pos ECEF4 : Scope
  Sat Position to VRML4 : Subsystem
  Out1 : Outport
  wires:
  Sat Position to VRML4/1(xVRML) -> Rate Transition11/1
  Rate Transition11/1 -> Out1/1
  In1/1 -> Sat Pos ECEF4/1, Sat Position to VRML4/1(x)

== system asbCubeSat.backup_210716a/Visualization/Virtual Reality World/Position conversion1 ==
  In1 : Inport
  Rate Transition11 : RateTransition
  Sat Pos ECEF4 : Scope
  Sat Position to VRML4 : Subsystem
  Out1 : Outport
  wires:
  Sat Position to VRML4/1(xVRML) -> Rate Transition11/1
  Rate Transition11/1 -> Out1/1
  In1/1 -> Sat Pos ECEF4/1, Sat Position to VRML4/1(x)

== system asbCubeSat.backup_210716a/Visualization/Virtual Reality World/Position conversion2 ==
  In1 : Inport
  Rate Transition11 : RateTransition
  Sat Pos ECEF4 : Scope
  Sat Position to VRML4 : Subsystem
  Out1 : Outport
  wires:
  Sat Position to VRML4/1(xVRML) -> Rate Transition11/1
  Rate Transition11/1 -> Out1/1
  In1/1 -> Sat Pos ECEF4/1, Sat Position to VRML4/1(x)

== system asbCubeSat.backup_210716a/Visualization/Virtual Reality World/Position conversion3 ==
  In1 : Inport
  Rate Transition11 : RateTransition
  Sat Pos ECEF4 : Scope
  Sat Position to VRML4 : Subsystem
  Out1 : Outport
  wires:
  Sat Position to VRML4/1(xVRML) -> Rate Transition11/1
  Rate Transition11/1 -> Out1/1
  In1/1 -> Sat Pos ECEF4/1, Sat Position to VRML4/1(x)

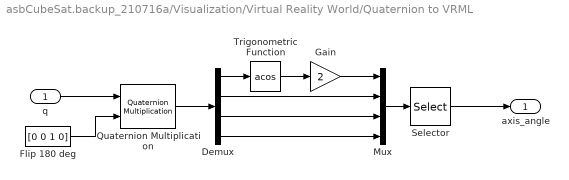
== system asbCubeSat.backup_210716a/Visualization/Virtual Reality World/Quaternion to VRML ==
  q : Inport
  Demux : Demux
  Flip 180 deg : Constant  Value=[0 0 1 0]
  Gain : Gain  Gain=2
  Mux : Mux
  Quaternion Multiplication : aerolibutil/Quaternion Multiplication
  Selector : Selector  InputPortWidth=4  IndexOptions=Index vector (dialog)  Indices=[3 4 2 1]  OutputSizes=1
  Trigonometric Function : Trigonometry  Operator=acos
  axis_angle : Outport  VectorParamsAs1DForOutWhenUnconnected=off
  wires:
  Demux/4 -> Mux/4
  Demux/3 -> Mux/3
  Demux/2 -> Mux/2
  Gain/1 -> Mux/1
  Selector/1 -> axis_angle/1
  q/1 -> Quaternion Multiplication/1
  Mux/1 -> Selector/1
  Trigonometric Function/1 -> Gain/1
  Demux/1 -> Trigonometric Function/1
  Flip 180 deg/1 -> Quaternion Multiplication/2
  Quaternion Multiplication/1 -> Demux/1

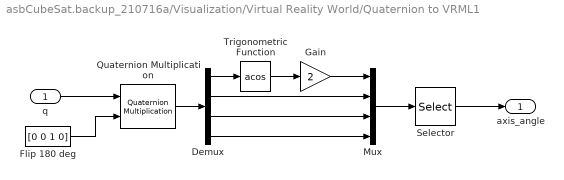
== system asbCubeSat.backup_210716a/Visualization/Virtual Reality World/Quaternion to VRML1 ==
  q : Inport
  Demux : Demux
  Flip 180 deg : Constant  Value=[0 0 1 0]
  Gain : Gain  Gain=2
  Mux : Mux
  Quaternion Multiplication : aerolibutil/Quaternion Multiplication
  Selector : Selector  InputPortWidth=4  IndexOptions=Index vector (dialog)  Indices=[3 4 2 1]  OutputSizes=1
  Trigonometric Function : Trigonometry  Operator=acos
  axis_angle : Outport  VectorParamsAs1DForOutWhenUnconnected=off
  wires:
  Demux/4 -> Mux/4
  Demux/3 -> Mux/3
  Demux/2 -> Mux/2
  Gain/1 -> Mux/1
  Selector/1 -> axis_angle/1
  Mux/1 -> Selector/1
  Trigonometric Function/1 -> Gain/1
  Demux/1 -> Trigonometric Function/1
  Flip 180 deg/1 -> Quaternion Multiplication/2
  q/1 -> Quaternion Multiplication/1
  Quaternion Multiplication/1 -> Demux/1

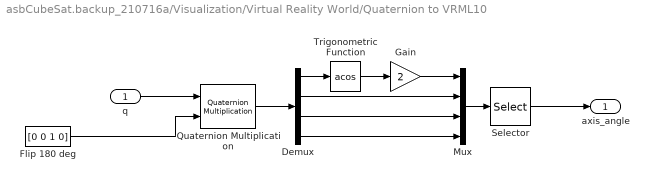
== system asbCubeSat.backup_210716a/Visualization/Virtual Reality World/Quaternion to VRML10 ==
  q : Inport
  Demux : Demux
  Flip 180 deg : Constant  Value=[0 0 1 0]
  Gain : Gain  Gain=2
  Mux : Mux
  Quaternion Multiplication : aerolibutil/Quaternion Multiplication
  Selector : Selector  InputPortWidth=4  IndexOptions=Index vector (dialog)  Indices=[3 4 2 1]  OutputSizes=1
  Trigonometric Function : Trigonometry  Operator=acos
  axis_angle : Outport  VectorParamsAs1DForOutWhenUnconnected=off
  wires:
  Demux/4 -> Mux/4
  Demux/3 -> Mux/3
  Demux/2 -> Mux/2
  Gain/1 -> Mux/1
  Selector/1 -> axis_angle/1
  Mux/1 -> Selector/1
  Trigonometric Function/1 -> Gain/1
  Demux/1 -> Trigonometric Function/1
  Flip 180 deg/1 -> Quaternion Multiplication/2
  q/1 -> Quaternion Multiplication/1
  Quaternion Multiplication/1 -> Demux/1

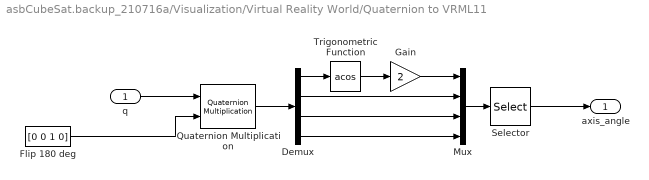
== system asbCubeSat.backup_210716a/Visualization/Virtual Reality World/Quaternion to VRML11 ==
  q : Inport
  Demux : Demux
  Flip 180 deg : Constant  Value=[0 0 1 0]
  Gain : Gain  Gain=2
  Mux : Mux
  Quaternion Multiplication : aerolibutil/Quaternion Multiplication
  Selector : Selector  InputPortWidth=4  IndexOptions=Index vector (dialog)  Indices=[3 4 2 1]  OutputSizes=1
  Trigonometric Function : Trigonometry  Operator=acos
  axis_angle : Outport  VectorParamsAs1DForOutWhenUnconnected=off
  wires:
  Demux/4 -> Mux/4
  Demux/3 -> Mux/3
  Demux/2 -> Mux/2
  Gain/1 -> Mux/1
  Selector/1 -> axis_angle/1
  Mux/1 -> Selector/1
  Trigonometric Function/1 -> Gain/1
  Demux/1 -> Trigonometric Function/1
  Flip 180 deg/1 -> Quaternion Multiplication/2
  q/1 -> Quaternion Multiplication/1
  Quaternion Multiplication/1 -> Demux/1

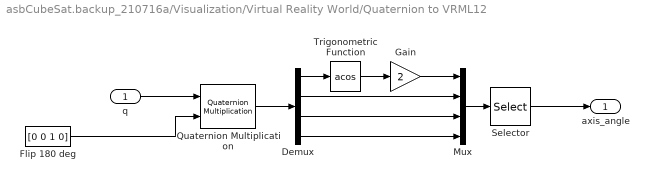
== system asbCubeSat.backup_210716a/Visualization/Virtual Reality World/Quaternion to VRML12 ==
  q : Inport
  Demux : Demux
  Flip 180 deg : Constant  Value=[0 0 1 0]
  Gain : Gain  Gain=2
  Mux : Mux
  Quaternion Multiplication : aerolibutil/Quaternion Multiplication
  Selector : Selector  InputPortWidth=4  IndexOptions=Index vector (dialog)  Indices=[3 4 2 1]  OutputSizes=1
  Trigonometric Function : Trigonometry  Operator=acos
  axis_angle : Outport  VectorParamsAs1DForOutWhenUnconnected=off
  wires:
  Demux/4 -> Mux/4
  Demux/3 -> Mux/3
  Demux/2 -> Mux/2
  Gain/1 -> Mux/1
  Selector/1 -> axis_angle/1
  Mux/1 -> Selector/1
  Trigonometric Function/1 -> Gain/1
  Demux/1 -> Trigonometric Function/1
  Flip 180 deg/1 -> Quaternion Multiplication/2
  q/1 -> Quaternion Multiplication/1
  Quaternion Multiplication/1 -> Demux/1

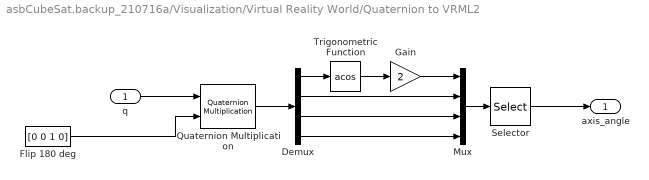
== system asbCubeSat.backup_210716a/Visualization/Virtual Reality World/Quaternion to VRML2 ==
  q : Inport
  Demux : Demux
  Flip 180 deg : Constant  Value=[0 0 1 0]
  Gain : Gain  Gain=2
  Mux : Mux
  Quaternion Multiplication : aerolibutil/Quaternion Multiplication
  Selector : Selector  InputPortWidth=4  IndexOptions=Index vector (dialog)  Indices=[3 4 2 1]  OutputSizes=1
  Trigonometric Function : Trigonometry  Operator=acos
  axis_angle : Outport  VectorParamsAs1DForOutWhenUnconnected=off
  wires:
  Demux/4 -> Mux/4
  Demux/3 -> Mux/3
  Demux/2 -> Mux/2
  Gain/1 -> Mux/1
  Selector/1 -> axis_angle/1
  q/1 -> Quaternion Multiplication/1
  Mux/1 -> Selector/1
  Trigonometric Function/1 -> Gain/1
  Demux/1 -> Trigonometric Function/1
  Flip 180 deg/1 -> Quaternion Multiplication/2
  Quaternion Multiplication/1 -> Demux/1

== system asbCubeSat.backup_210716a/Visualization/Virtual Reality World/Quaternion to VRML9 ==
  q : Inport
  Demux : Demux
  Flip 180 deg : Constant  Value=[0 0 1 0]
  Gain : Gain  Gain=2
  Mux : Mux
  Quaternion Multiplication : aerolibutil/Quaternion Multiplication
  Selector : Selector  InputPortWidth=4  IndexOptions=Index vector (dialog)  Indices=[3 4 2 1]  OutputSizes=1
  Trigonometric Function : Trigonometry  Operator=acos
  axis_angle : Outport  VectorParamsAs1DForOutWhenUnconnected=off
  wires:
  Demux/4 -> Mux/4
  Demux/3 -> Mux/3
  Demux/2 -> Mux/2
  Gain/1 -> Mux/1
  Selector/1 -> axis_angle/1
  Mux/1 -> Selector/1
  Trigonometric Function/1 -> Gain/1
  Demux/1 -> Trigonometric Function/1
  Flip 180 deg/1 -> Quaternion Multiplication/2
  q/1 -> Quaternion Multiplication/1
  Quaternion Multiplication/1 -> Demux/1

== system asbCubeSat.backup_210716a/Visualization/Virtual Reality World/Radar on//off ==
  NavMode : Inport
  Add : Sum  Inputs=-+
  Compare To Constant : simulink/Logic and Bit Operations/Compare To Constant  relop===  const=1  OutDataTypeStr=boolean  ZeroCross=off
  Constant : Constant
  Data Type Conversion : DataTypeConversion  OutDataTypeStr=double
  Gain : Gain  Gain=0.6
  Radar : Outport  VectorParamsAs1DForOutWhenUnconnected=off
  wires:
  NavMode/1 -> Compare To Constant/1
  Compare To Constant/1 -> Data Type Conversion/1
  Data Type Conversion/1 -> Gain/1
  Gain/1 -> Add/1
  Constant/1 -> Add/2
  Add/1 -> Radar/1

== system asbCubeSat.backup_210716a/Visualization/Virtual Reality World/Sat Position to VRML ==
  x : Inport
  ECEF to VRML : Subsystem
  Length Conversion : aerolibconvert2/Length Conversion  IU=m  OU=km
  km to VRML units : Gain  Gain=1/1000
  xVRML : Outport  VectorParamsAs1DForOutWhenUnconnected=off
  wires:
  ECEF to VRML/1(VR) -> xVRML/1
  x/1 -> Length Conversion/1
  km to VRML units/1 -> ECEF to VRML/1(M)
  Length Conversion/1 -> km to VRML units/1

== system asbCubeSat.backup_210716a/Visualization/Virtual Reality World/Satellite Model Scaling ==
  Constant : Constant  Value=cubesatSize
  Mux : Mux  Inputs=3
  ScaleModelToVRML : Gain  Gain=1/.3e6
  ScaleModelToVRML1 : Gain  Gain=1/10
  Out1 : Outport  VectorParamsAs1DForOutWhenUnconnected=off
  wires:
  ScaleModelToVRML/1 -> Mux/3, Mux/1, Mux/2
  Mux/1 -> Out1/1
  Constant/1 -> ScaleModelToVRML1/1
  ScaleModelToVRML1/1 -> ScaleModelToVRML/1

== system asbCubeSat.backup_210716a/Visualization/Virtual Reality World/Sun Position to VRML ==
  x : Inport
  ECEF to VRML : Subsystem
  Length Conversion : aerolibconvert2/Length Conversion  IU=m  OU=km
  km to VRML units : Gain  Gain=1/1000
  xVRML : Outport  VectorParamsAs1DForOutWhenUnconnected=off
  wires:
  ECEF to VRML/1(VR) -> xVRML/1
  x/1 -> Length Conversion/1
  km to VRML units/1 -> ECEF to VRML/1(M)
  Length Conversion/1 -> km to VRML units/1

== system asbCubeSat.backup_210716a/Visualization/Virtual Reality World/Antenna Position to VRML/ECEF to VRML ==
  M : Inport  PortDimensions=3
  Selector : Selector  InputPortWidth=3  IndexOptions=Index vector (dialog)  Indices=[2 3 1]  OutputSizes=1
  VR : Outport  PortDimensions=3  VectorParamsAs1DForOutWhenUnconnected=off
  wires:
  M/1 -> Selector/1
  Selector/1 -> VR/1

== system asbCubeSat.backup_210716a/Visualization/Virtual Reality World/Compute Earth Rotation Rate/Quaternion to VRML ==
  q : Inport
  Demux : Demux
  Gain : Gain  Gain=2
  Gain3 : Gain  Gain=[-1 1 1 1]
  Mux : Mux
  Selector : Selector  InputPortWidth=4  IndexOptions=Index vector (dialog)  Indices=[2 4 3 1]  OutputSizes=1
  Trigonometric Function : Trigonometry  Operator=acos
  AxisAngle : Outport  VectorParamsAs1DForOutWhenUnconnected=off
  wires:
  Demux/4 -> Mux/4
  Demux/3 -> Mux/3
  Demux/2 -> Mux/2
  Gain/1 -> Mux/1
  Selector/1 -> Gain3/1
  Gain3/1 -> AxisAngle/1
  q/1 -> Demux/1
  Mux/1 -> Selector/1
  Trigonometric Function/1 -> Gain/1
  Demux/1 -> Trigonometric Function/1

== system asbCubeSat.backup_210716a/Visualization/Virtual Reality World/Compute Umbra Translation/unitVec ==
  I : Inport
  Divide : Product  Inputs=*/
  Dot Product : DotProduct  InputSameDT=on  OutDataTypeStr=Inherit: Inherit via internal rule
  Sqrt : Sqrt  SaturateOnIntegerOverflow=on
  O : Outport  VectorParamsAs1DForOutWhenUnconnected=off
  wires:
  Dot Product/1 -> Sqrt/1
  I/1 -> Divide/1, Dot Product/1, Dot Product/2
  Divide/1 -> O/1
  Sqrt/1 -> Divide/2

== system asbCubeSat.backup_210716a/Visualization/Virtual Reality World/Position conversion4/Sat Position to VRML4 ==
  x : Inport
  ECEF to VRML : Subsystem
  Length Conversion : aerolibconvert2/Length Conversion  IU=m  OU=km
  km to VRML units : Gain  Gain=1/1000
  xVRML : Outport  VectorParamsAs1DForOutWhenUnconnected=off
  wires:
  ECEF to VRML/1(VR) -> xVRML/1
  x/1 -> Length Conversion/1
  km to VRML units/1 -> ECEF to VRML/1(M)
  Length Conversion/1 -> km to VRML units/1

== system asbCubeSat.backup_210716a/Visualization/Virtual Reality World/Position conversion1/Sat Position to VRML4 ==
  x : Inport
  ECEF to VRML : Subsystem
  Length Conversion : aerolibconvert2/Length Conversion  IU=m  OU=km
  km to VRML units : Gain  Gain=1/1000
  xVRML : Outport  VectorParamsAs1DForOutWhenUnconnected=off
  wires:
  ECEF to VRML/1(VR) -> xVRML/1
  x/1 -> Length Conversion/1
  km to VRML units/1 -> ECEF to VRML/1(M)
  Length Conversion/1 -> km to VRML units/1

== system asbCubeSat.backup_210716a/Visualization/Virtual Reality World/Position conversion2/Sat Position to VRML4 ==
  x : Inport
  ECEF to VRML : Subsystem
  Length Conversion : aerolibconvert2/Length Conversion  IU=m  OU=km
  km to VRML units : Gain  Gain=1/1000
  xVRML : Outport  VectorParamsAs1DForOutWhenUnconnected=off
  wires:
  ECEF to VRML/1(VR) -> xVRML/1
  x/1 -> Length Conversion/1
  km to VRML units/1 -> ECEF to VRML/1(M)
  Length Conversion/1 -> km to VRML units/1

== system asbCubeSat.backup_210716a/Visualization/Virtual Reality World/Position conversion3/Sat Position to VRML4 ==
  x : Inport
  ECEF to VRML : Subsystem
  Length Conversion : aerolibconvert2/Length Conversion  IU=m  OU=km
  km to VRML units : Gain  Gain=1/1000
  xVRML : Outport  VectorParamsAs1DForOutWhenUnconnected=off
  wires:
  ECEF to VRML/1(VR) -> xVRML/1
  x/1 -> Length Conversion/1
  km to VRML units/1 -> ECEF to VRML/1(M)
  Length Conversion/1 -> km to VRML units/1

== system asbCubeSat.backup_210716a/Visualization/Virtual Reality World/Sat Position to VRML/ECEF to VRML ==
  M : Inport  PortDimensions=3
  Selector : Selector  InputPortWidth=3  IndexOptions=Index vector (dialog)  Indices=[2 3 1]  OutputSizes=1
  VR : Outport  PortDimensions=3  VectorParamsAs1DForOutWhenUnconnected=off
  wires:
  M/1 -> Selector/1
  Selector/1 -> VR/1

== system asbCubeSat.backup_210716a/Visualization/Virtual Reality World/Sun Position to VRML/ECEF to VRML ==
  M : Inport  PortDimensions=3
  Selector : Selector  InputPortWidth=3  IndexOptions=Index vector (dialog)  Indices=[2 3 1]  OutputSizes=1
  VR : Outport  PortDimensions=3  VectorParamsAs1DForOutWhenUnconnected=off
  wires:
  M/1 -> Selector/1
  Selector/1 -> VR/1

== system asbCubeSat.backup_210716a/Visualization/Virtual Reality World/Position conversion4/Sat Position to VRML4/ECEF to VRML ==
  M : Inport  PortDimensions=3
  Selector : Selector  InputPortWidth=3  IndexOptions=Index vector (dialog)  Indices=[2 3 1]  OutputSizes=1
  VR : Outport  PortDimensions=3  VectorParamsAs1DForOutWhenUnconnected=off
  wires:
  M/1 -> Selector/1
  Selector/1 -> VR/1

== system asbCubeSat.backup_210716a/Visualization/Virtual Reality World/Position conversion1/Sat Position to VRML4/ECEF to VRML ==
  M : Inport  PortDimensions=3
  Selector : Selector  InputPortWidth=3  IndexOptions=Index vector (dialog)  Indices=[2 3 1]  OutputSizes=1
  VR : Outport  PortDimensions=3  VectorParamsAs1DForOutWhenUnconnected=off
  wires:
  M/1 -> Selector/1
  Selector/1 -> VR/1

== system asbCubeSat.backup_210716a/Visualization/Virtual Reality World/Position conversion2/Sat Position to VRML4/ECEF to VRML ==
  M : Inport  PortDimensions=3
  Selector : Selector  InputPortWidth=3  IndexOptions=Index vector (dialog)  Indices=[2 3 1]  OutputSizes=1
  VR : Outport  PortDimensions=3  VectorParamsAs1DForOutWhenUnconnected=off
  wires:
  M/1 -> Selector/1
  Selector/1 -> VR/1

== system asbCubeSat.backup_210716a/Visualization/Virtual Reality World/Position conversion3/Sat Position to VRML4/ECEF to VRML ==
  M : Inport  PortDimensions=3
  Selector : Selector  InputPortWidth=3  IndexOptions=Index vector (dialog)  Indices=[2 3 1]  OutputSizes=1
  VR : Outport  PortDimensions=3  VectorParamsAs1DForOutWhenUnconnected=off
  wires:
  M/1 -> Selector/1
  Selector/1 -> VR/1
